simulink model "Symulacje"  (R2022a)
settings: Solver=VariableStepAuto  StartTime=0.0  StopTime=10000.0  RelTol=0.000001
undefined symbols (not defined in the file): aG1, aG2, aM1, aM2, aM3, aP1, aP2, aP3, bG1, bG2, bM1, bM2, bM3, bP1, bP2, bP3, cG1, cG2, cM1, cM2, cM3, cP1, cP2, cP3, DiscIntNeverNeededParam, KG1, KG2, KG3, KM1, KM2, KM3, KP1, KP2, KP3, kr1, kr2, kr3, T01, T02, T03, TG32, Ti1, Ti2, Ti3, Tzad1, Tzad2, Tzad3, waga1, waga2, waga3, waga4, waga5, waga6, waga7, waga8, waga9
libraries: simulink x15
settings Model: Creator=zawod  LastModifiedBy=zawod
settings SolverCC: ZeroCrossAlgorithm=Adaptive
settings DebuggingCC: AlgebraicLoopMsg=none  IgnoredZcDiagnostic=none

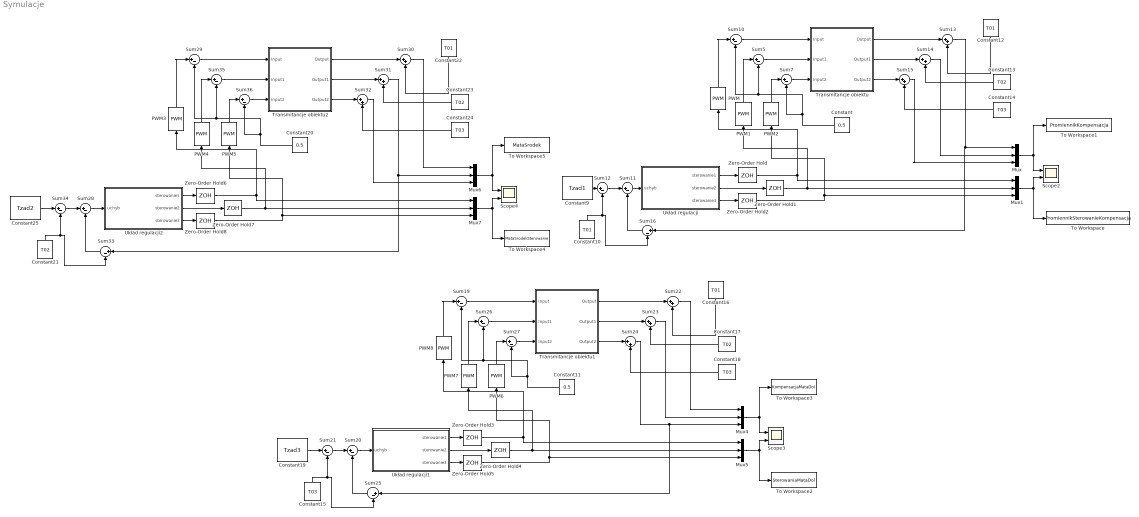
== system Symulacje ==
  Constant : Constant  Value=0.5
  Constant{10,12,16,22} (4 alike) : Constant  Value=T01
  Constant11 : Constant  Value=0.5
  Constant{13,17,21,23} (4 alike) : Constant  Value=T02
  Constant{14..15,18,24} (4 alike) : Constant  Value=T03
  Constant19 : Constant  Value=Tzad3
  Constant20 : Constant  Value=0.5
  Constant25 : Constant  Value=Tzad2
  Constant9 : Constant  Value=Tzad1
  Mux{,1,4..7} (6 alike) : Mux  Inputs=3
  PWM{,1..8} (9 alike) : simulink/Discontinuities/PWM  DisableCoverage=on  Period=10  DisallowZeroDutyCycle=off  RunAtFixedTimeIntervals=off  SampleTime=0.1
  Scope2 : Scope  NumInputPorts=2
  Scope3 : Scope  NumInputPorts=2
  Scope4 : Scope  NumInputPorts=2
  Sum{5,7,10..12,16,19..21,25..29,33..36} (18 alike) : Sum  Inputs=|+-
  Sum{13..15,22..24,30..32} (9 alike) : Sum  Inputs=|++
  To Workspace : ToWorkspace  VariableName=PromiennikSterowanieKompensacja  SaveFormat=Timeseries  SampleTime=-1
  To Workspace1 : ToWorkspace  VariableName=PromiennikKompensacja  SaveFormat=Timeseries  SampleTime=-1
  To Workspace2 : ToWorkspace  VariableName=SterowaniaMataDol  SaveFormat=Timeseries  SampleTime=-1
  To Workspace3 : ToWorkspace  VariableName=KompensacjaMataDol  SaveFormat=Timeseries  SampleTime=-1
  To Workspace4 : ToWorkspace  VariableName=MataSrodekSterowanie  SaveFormat=Timeseries  SampleTime=-1
  To Workspace5 : ToWorkspace  VariableName=MataSrodek  SaveFormat=Timeseries  SampleTime=-1
  Transmitancje obiektu : Subsystem
  Transmitancje obiektu1 : Subsystem
  Transmitancje obiektu2 : Subsystem
  Układ regulacji : Subsystem  mask{Kr=kr1, Ti=Ti1, Max=0.5, Min=-0.5}
      mask prompts: Kr "Kp"
  Układ regulacji1 : Subsystem  mask{Kr=kr3, Ti=Ti3, Max=0.5, Min=-0.5}
      mask prompts: Kr "Kp"
  Układ regulacji2 : Subsystem  mask{Kr=kr2, Ti=Ti2, Max=0.5, Min=-0.5}
      mask prompts: Kr "Kp"
  Zero-Order Hold{,1..8} (9 alike) : ZeroOrderHold  SampleTime=30
  wires:
  Transmitancje obiektu/3(Output2) -> Sum15/1
  Układ regulacji/3(sterowanie3) -> Zero-Order Hold2/1
  Constant/1 -> Sum10/2, Sum5/2, Sum7/2
  Constant9/1 -> Sum12/1
  Mux1/1 -> To Workspace/1, Scope2/2
  Constant13/1 -> Sum14/2
  Mux/1 -> Scope2/1, To Workspace1/1
  Układ regulacji/1(sterowanie1) -> Zero-Order Hold/1
  Układ regulacji/2(sterowanie2) -> Zero-Order Hold1/1
  Transmitancje obiektu/1(Output) -> Sum13/1
  Sum11/1 -> Układ regulacji/1(uchyb)
  Sum12/1 -> Sum11/1
  Constant12/1 -> Sum13/2
  Sum10/1 -> Transmitancje obiektu/1(Input)
  Constant10/1 -> Sum16/2, Sum12/2
  Sum16/1 -> Sum11/2
  Constant14/1 -> Sum15/2
  Transmitancje obiektu/2(Output1) -> Sum14/1
  Sum7/1 -> Transmitancje obiektu/3(Input2)
  Sum5/1 -> Transmitancje obiektu/2(Input1)
  Zero-Order Hold/1 -> PWM/1, Mux1/1
  Zero-Order Hold1/1 -> PWM1/1, Mux1/2
  Zero-Order Hold2/1 -> Mux1/3, PWM2/1
  Sum14/1 -> Mux/2
  Sum15/1 -> Mux/3
  Constant18/1 -> Sum24/2
  Sum20/1 -> Układ regulacji1/1(uchyb)
  Transmitancje obiektu1/2(Output1) -> Sum23/1
  Transmitancje obiektu1/3(Output2) -> Sum24/1
  Constant16/1 -> Sum22/2
  Sum27/1 -> Transmitancje obiektu1/3(Input2)
  Układ regulacji1/1(sterowanie1) -> Zero-Order Hold3/1
  Mux5/1 -> To Workspace2/1, Scope3/2
  Zero-Order Hold4/1 -> PWM7/1, Mux5/2
  Sum26/1 -> Transmitancje obiektu1/2(Input1)
  Zero-Order Hold3/1 -> PWM8/1, Mux5/1
  Sum22/1 -> Mux4/1
  Sum23/1 -> Mux4/2
  Constant15/1 -> Sum25/2, Sum21/2
  Sum19/1 -> Transmitancje obiektu1/1(Input)
  Constant11/1 -> Sum26/2, Sum19/2, Sum27/2
  Constant19/1 -> Sum21/1
  Constant17/1 -> Sum23/2
  Mux4/1 -> Scope3/1, To Workspace3/1
  Transmitancje obiektu1/1(Output) -> Sum22/1
  Układ regulacji1/3(sterowanie3) -> Zero-Order Hold5/1
  Zero-Order Hold5/1 -> Mux5/3, PWM6/1
  Sum25/1 -> Sum20/2
  Układ regulacji1/2(sterowanie2) -> Zero-Order Hold4/1
  Sum21/1 -> Sum20/1
  Sum30/1 -> Mux6/1
  Mux7/1 -> To Workspace4/1, Scope4/2
  Sum33/1 -> Sum28/2
  Mux6/1 -> Scope4/1, To Workspace5/1
  Constant22/1 -> Sum30/2
  Sum29/1 -> Transmitancje obiektu2/1(Input)
  Transmitancje obiektu2/3(Output2) -> Sum32/1
  Sum34/1 -> Sum28/1
  Constant24/1 -> Sum32/2
  Układ regulacji2/2(sterowanie2) -> Zero-Order Hold7/1
  Transmitancje obiektu2/2(Output1) -> Sum31/1
  Constant20/1 -> Sum35/2, Sum29/2, Sum36/2
  Transmitancje obiektu2/1(Output) -> Sum30/1
  Sum28/1 -> Układ regulacji2/1(uchyb)
  Zero-Order Hold6/1 -> PWM3/1, Mux7/1
  Sum35/1 -> Transmitancje obiektu2/2(Input1)
  Sum32/1 -> Mux6/3
  Układ regulacji2/3(sterowanie3) -> Zero-Order Hold8/1
  Sum36/1 -> Transmitancje obiektu2/3(Input2)
  Zero-Order Hold8/1 -> Mux7/3, PWM5/1
  Constant25/1 -> Sum34/1
  Constant23/1 -> Sum31/2
  Zero-Order Hold7/1 -> PWM4/1, Mux7/2
  Układ regulacji2/1(sterowanie1) -> Zero-Order Hold6/1
  Constant21/1 -> Sum33/2, Sum34/2
  PWM/1 -> Sum10/1
  PWM1/1 -> Sum5/1
  PWM2/1 -> Sum7/1
  Sum13/1 -> Sum16/1, Mux/1
  Sum24/1 -> Sum25/1, Mux4/3
  Sum31/1 -> Sum33/1, Mux6/2
  PWM3/1 -> Sum29/1
  PWM4/1 -> Sum35/1
  PWM5/1 -> Sum36/1
  PWM6/1 -> Sum27/1
  PWM7/1 -> Sum26/1
  PWM8/1 -> Sum19/1

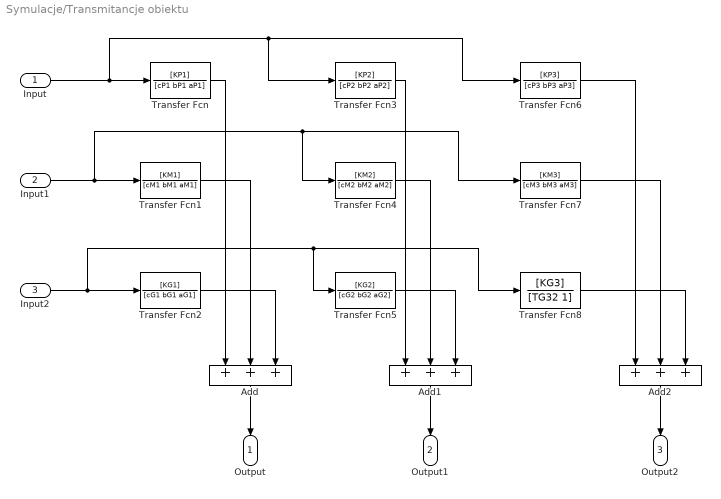
== system Symulacje/Transmitancje obiektu ==
  Input : Inport
  Input1 : Inport  Port=2
  Input2 : Inport  Port=3
  Add : Sum  Inputs=+++
  Add1 : Sum  Inputs=+++
  Add2 : Sum  Inputs=+++
  Transfer Fcn : TransferFcn  Numerator=[KP1]  Denominator=[cP1 bP1 aP1]
  Transfer Fcn1 : TransferFcn  Numerator=[KM1]  Denominator=[cM1 bM1 aM1]
  Transfer Fcn2 : TransferFcn  Numerator=[KG1]  Denominator=[cG1 bG1 aG1]
  Transfer Fcn3 : TransferFcn  Numerator=[KP2]  Denominator=[cP2 bP2 aP2]
  Transfer Fcn4 : TransferFcn  Numerator=[KM2]  Denominator=[cM2 bM2 aM2]
  Transfer Fcn5 : TransferFcn  Numerator=[KG2]  Denominator=[cG2 bG2 aG2]
  Transfer Fcn6 : TransferFcn  Numerator=[KP3]  Denominator=[cP3 bP3 aP3]
  Transfer Fcn7 : TransferFcn  Numerator=[KM3]  Denominator=[cM3 bM3 aM3]
  Transfer Fcn8 : TransferFcn  Numerator=[KG3]  Denominator=[TG32 1]
  Output : Outport
  Output1 : Outport  Port=2
  Output2 : Outport  Port=3
  wires:
  Input2/1 -> Transfer Fcn5/1, Transfer Fcn8/1, Transfer Fcn2/1
  Add1/1 -> Output1/1
  Transfer Fcn3/1 -> Add1/1
  Input1/1 -> Transfer Fcn7/1, Transfer Fcn4/1, Transfer Fcn1/1
  Transfer Fcn4/1 -> Add1/2
  Transfer Fcn8/1 -> Add2/3
  Transfer Fcn6/1 -> Add2/1
  Transfer Fcn5/1 -> Add1/3
  Add/1 -> Output/1
  Add2/1 -> Output2/1
  Transfer Fcn1/1 -> Add/2
  Transfer Fcn2/1 -> Add/3
  Input/1 -> Transfer Fcn6/1, Transfer Fcn3/1, Transfer Fcn/1
  Transfer Fcn/1 -> Add/1
  Transfer Fcn7/1 -> Add2/2

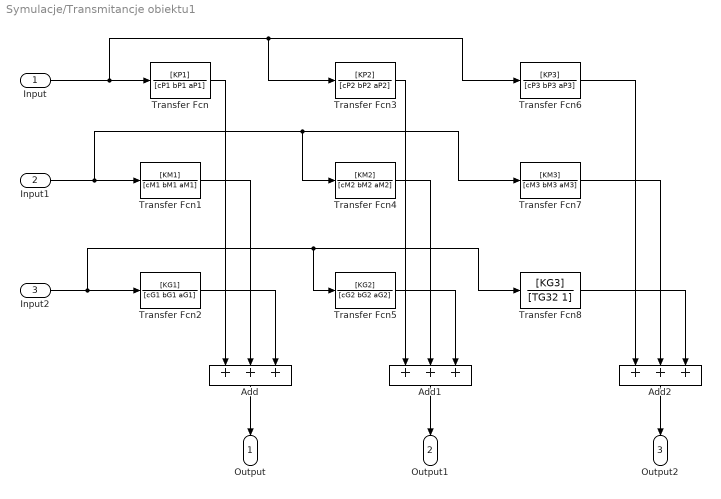
== system Symulacje/Transmitancje obiektu1 ==
  Input : Inport
  Input1 : Inport  Port=2
  Input2 : Inport  Port=3
  Add : Sum  Inputs=+++
  Add1 : Sum  Inputs=+++
  Add2 : Sum  Inputs=+++
  Transfer Fcn : TransferFcn  Numerator=[KP1]  Denominator=[cP1 bP1 aP1]
  Transfer Fcn1 : TransferFcn  Numerator=[KM1]  Denominator=[cM1 bM1 aM1]
  Transfer Fcn2 : TransferFcn  Numerator=[KG1]  Denominator=[cG1 bG1 aG1]
  Transfer Fcn3 : TransferFcn  Numerator=[KP2]  Denominator=[cP2 bP2 aP2]
  Transfer Fcn4 : TransferFcn  Numerator=[KM2]  Denominator=[cM2 bM2 aM2]
  Transfer Fcn5 : TransferFcn  Numerator=[KG2]  Denominator=[cG2 bG2 aG2]
  Transfer Fcn6 : TransferFcn  Numerator=[KP3]  Denominator=[cP3 bP3 aP3]
  Transfer Fcn7 : TransferFcn  Numerator=[KM3]  Denominator=[cM3 bM3 aM3]
  Transfer Fcn8 : TransferFcn  Numerator=[KG3]  Denominator=[TG32 1]
  Output : Outport
  Output1 : Outport  Port=2
  Output2 : Outport  Port=3
  wires:
  Input2/1 -> Transfer Fcn5/1, Transfer Fcn8/1, Transfer Fcn2/1
  Add1/1 -> Output1/1
  Transfer Fcn3/1 -> Add1/1
  Input1/1 -> Transfer Fcn7/1, Transfer Fcn4/1, Transfer Fcn1/1
  Transfer Fcn4/1 -> Add1/2
  Transfer Fcn8/1 -> Add2/3
  Transfer Fcn6/1 -> Add2/1
  Transfer Fcn5/1 -> Add1/3
  Add/1 -> Output/1
  Add2/1 -> Output2/1
  Transfer Fcn1/1 -> Add/2
  Transfer Fcn2/1 -> Add/3
  Input/1 -> Transfer Fcn6/1, Transfer Fcn3/1, Transfer Fcn/1
  Transfer Fcn/1 -> Add/1
  Transfer Fcn7/1 -> Add2/2

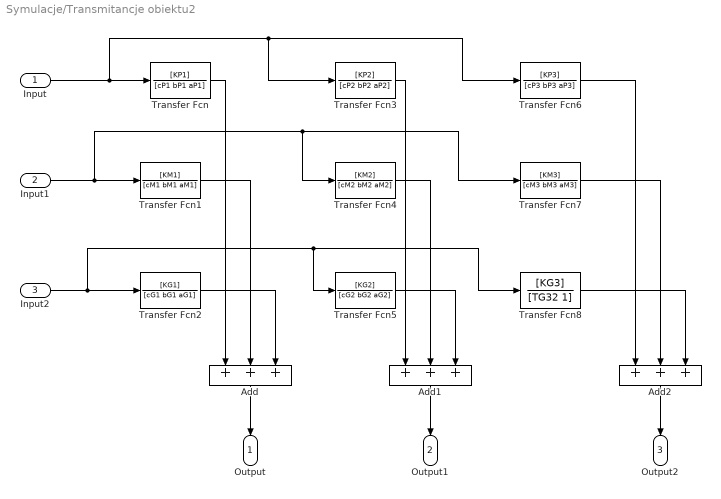
== system Symulacje/Transmitancje obiektu2 ==
  Input : Inport
  Input1 : Inport  Port=2
  Input2 : Inport  Port=3
  Add : Sum  Inputs=+++
  Add1 : Sum  Inputs=+++
  Add2 : Sum  Inputs=+++
  Transfer Fcn : TransferFcn  Numerator=[KP1]  Denominator=[cP1 bP1 aP1]
  Transfer Fcn1 : TransferFcn  Numerator=[KM1]  Denominator=[cM1 bM1 aM1]
  Transfer Fcn2 : TransferFcn  Numerator=[KG1]  Denominator=[cG1 bG1 aG1]
  Transfer Fcn3 : TransferFcn  Numerator=[KP2]  Denominator=[cP2 bP2 aP2]
  Transfer Fcn4 : TransferFcn  Numerator=[KM2]  Denominator=[cM2 bM2 aM2]
  Transfer Fcn5 : TransferFcn  Numerator=[KG2]  Denominator=[cG2 bG2 aG2]
  Transfer Fcn6 : TransferFcn  Numerator=[KP3]  Denominator=[cP3 bP3 aP3]
  Transfer Fcn7 : TransferFcn  Numerator=[KM3]  Denominator=[cM3 bM3 aM3]
  Transfer Fcn8 : TransferFcn  Numerator=[KG3]  Denominator=[TG32 1]
  Output : Outport
  Output1 : Outport  Port=2
  Output2 : Outport  Port=3
  wires:
  Input2/1 -> Transfer Fcn5/1, Transfer Fcn8/1, Transfer Fcn2/1
  Add1/1 -> Output1/1
  Transfer Fcn3/1 -> Add1/1
  Input1/1 -> Transfer Fcn7/1, Transfer Fcn4/1, Transfer Fcn1/1
  Transfer Fcn4/1 -> Add1/2
  Transfer Fcn8/1 -> Add2/3
  Transfer Fcn6/1 -> Add2/1
  Transfer Fcn5/1 -> Add1/3
  Add/1 -> Output/1
  Add2/1 -> Output2/1
  Transfer Fcn1/1 -> Add/2
  Transfer Fcn2/1 -> Add/3
  Input/1 -> Transfer Fcn6/1, Transfer Fcn3/1, Transfer Fcn/1
  Transfer Fcn/1 -> Add/1
  Transfer Fcn7/1 -> Add2/2

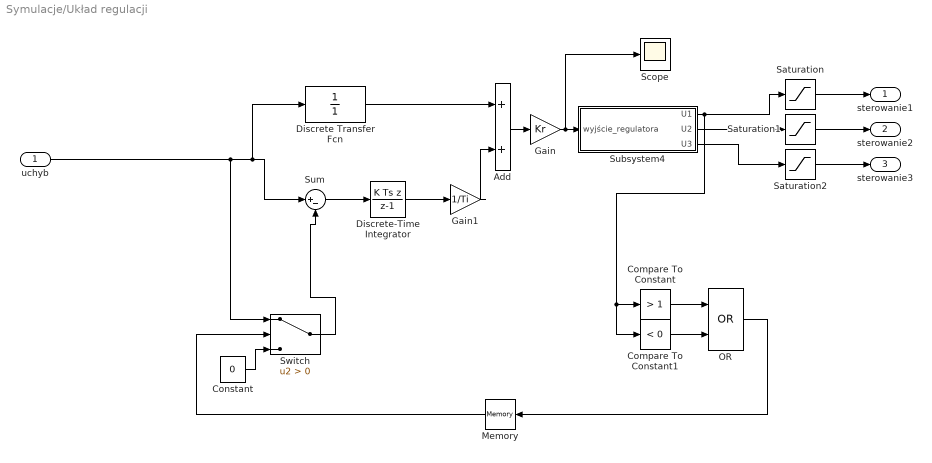
== system Symulacje/Układ regulacji ==
  uchyb : Inport
  Add : Sum
  Compare To Constant : simulink/Logic and Bit Operations/Compare To Constant  relop=>  const=1  OutDataTypeStr=uint8
  Compare To Constant1 : simulink/Logic and Bit Operations/Compare To Constant  relop=<  const=0  OutDataTypeStr=uint8
  Constant : Constant  Value=0
  Discrete Transfer Fcn : DiscreteTransferFcn  Denominator=[1]  SampleTime=30
  Discrete-Time Integrator : DiscreteIntegrator  IntegratorMethod=Integration: Backward Euler  SampleTime=30  ICPrevOutput=DiscIntNeverNeededParam  ICPrevScaledInput=DiscIntNeverNeededParam
  Gain : Gain  Gain=Kr
  Gain1 : Gain  Gain=1/Ti
  Memory : Memory
  OR : Logic  Operator=OR  IconShape=distinctive  AllPortsSameDT=off  OutDataTypeStr=boolean
  Saturation : Saturate  UpperLimit=1  LowerLimit=0
  Saturation1 : Saturate  UpperLimit=1  LowerLimit=0
  Saturation2 : Saturate  UpperLimit=1  LowerLimit=0
  Scope : Scope
  Subsystem4 : Subsystem
  Sum : Sum  Inputs=|+-
  Switch : Switch  Criteria=u2 > Threshold  SaturateOnIntegerOverflow=off  InputSameDT=off
  sterowanie1 : Outport
  sterowanie2 : Outport  Port=2
  sterowanie3 : Outport  Port=3
  wires:
  Gain1/1 -> Add/2
  Add/1 -> Gain/1
  Discrete-Time Integrator/1 -> Gain1/1
  Sum/1 -> Discrete-Time Integrator/1
  Switch/1 -> Sum/2
  Constant/1 -> Switch/3
  Subsystem4/2(U2) -> Saturation1/1
  Subsystem4/3(U3) -> Saturation2/1
  Subsystem4/1(U1) -> Saturation/1, Compare To Constant/1, Compare To Constant1/1
  Saturation/1 -> sterowanie1/1
  Saturation1/1 -> sterowanie2/1
  Saturation2/1 -> sterowanie3/1
  Compare To Constant/1 -> OR/1
  Compare To Constant1/1 -> OR/2
  Gain/1 -> Scope/1, Subsystem4/1(wyjście_regulatora)
  Memory/1 -> Switch/2
  uchyb/1 -> Sum/1, Discrete Transfer Fcn/1, Switch/1
  Discrete Transfer Fcn/1 -> Add/1
  OR/1 -> Memory/1

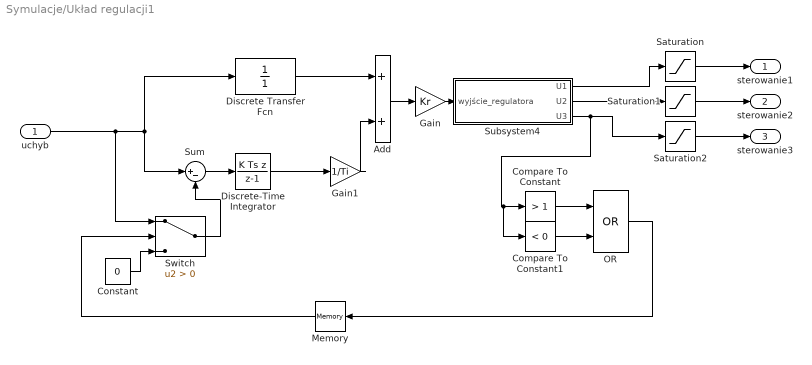
== system Symulacje/Układ regulacji1 ==
  uchyb : Inport
  Add : Sum
  Compare To Constant : simulink/Logic and Bit Operations/Compare To Constant  relop=>  const=1  OutDataTypeStr=boolean
  Compare To Constant1 : simulink/Logic and Bit Operations/Compare To Constant  relop=<  const=0  OutDataTypeStr=boolean
  Constant : Constant  Value=0
  Discrete Transfer Fcn : DiscreteTransferFcn  Denominator=[1]  SampleTime=30
  Discrete-Time Integrator : DiscreteIntegrator  IntegratorMethod=Integration: Backward Euler  SampleTime=30  ICPrevOutput=DiscIntNeverNeededParam  ICPrevScaledInput=DiscIntNeverNeededParam
  Gain : Gain  Gain=Kr
  Gain1 : Gain  Gain=1/Ti
  Memory : Memory
  OR : Logic  Operator=OR  IconShape=distinctive  AllPortsSameDT=off  OutDataTypeStr=boolean
  Saturation : Saturate  UpperLimit=1  LowerLimit=0
  Saturation1 : Saturate  UpperLimit=1  LowerLimit=0
  Saturation2 : Saturate  UpperLimit=1  LowerLimit=0
  Subsystem4 : Subsystem
  Sum : Sum  Inputs=|+-
  Switch : Switch  Criteria=u2 > Threshold  SaturateOnIntegerOverflow=off  InputSameDT=off
  sterowanie1 : Outport
  sterowanie2 : Outport  Port=2
  sterowanie3 : Outport  Port=3
  wires:
  Gain1/1 -> Add/2
  Add/1 -> Gain/1
  Discrete-Time Integrator/1 -> Gain1/1
  Sum/1 -> Discrete-Time Integrator/1
  Switch/1 -> Sum/2
  Constant/1 -> Switch/3
  Subsystem4/2(U2) -> Saturation1/1
  Subsystem4/3(U3) -> Compare To Constant1/1, Compare To Constant/1, Saturation2/1
  Gain/1 -> Subsystem4/1(wyjście_regulatora)
  Subsystem4/1(U1) -> Saturation/1
  Saturation/1 -> sterowanie1/1
  Saturation1/1 -> sterowanie2/1
  Saturation2/1 -> sterowanie3/1
  Compare To Constant/1 -> OR/1
  Compare To Constant1/1 -> OR/2
  OR/1 -> Memory/1
  uchyb/1 -> Switch/1, Sum/1, Discrete Transfer Fcn/1
  Memory/1 -> Switch/2
  Discrete Transfer Fcn/1 -> Add/1

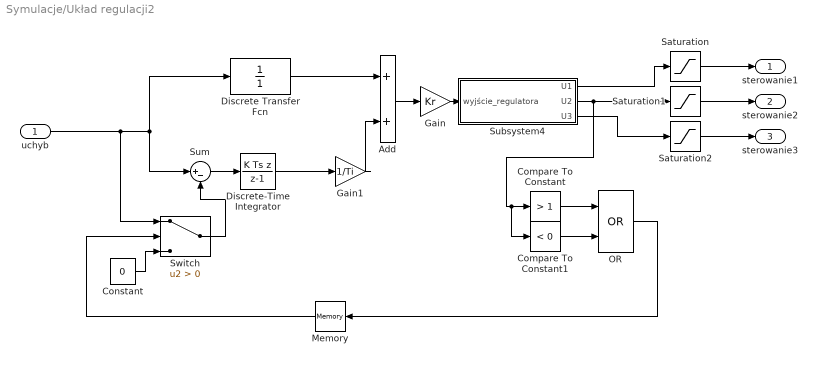
== system Symulacje/Układ regulacji2 ==
  uchyb : Inport
  Add : Sum
  Compare To Constant : simulink/Logic and Bit Operations/Compare To Constant  relop=>  const=1  OutDataTypeStr=boolean
  Compare To Constant1 : simulink/Logic and Bit Operations/Compare To Constant  relop=<  const=0  OutDataTypeStr=boolean
  Constant : Constant  Value=0
  Discrete Transfer Fcn : DiscreteTransferFcn  Denominator=[1]  SampleTime=30
  Discrete-Time Integrator : DiscreteIntegrator  IntegratorMethod=Integration: Backward Euler  SampleTime=30  ICPrevOutput=DiscIntNeverNeededParam  ICPrevScaledInput=DiscIntNeverNeededParam
  Gain : Gain  Gain=Kr
  Gain1 : Gain  Gain=1/Ti
  Memory : Memory
  OR : Logic  Operator=OR  IconShape=distinctive  AllPortsSameDT=off  OutDataTypeStr=boolean
  Saturation : Saturate  UpperLimit=1  LowerLimit=0
  Saturation1 : Saturate  UpperLimit=1  LowerLimit=0
  Saturation2 : Saturate  UpperLimit=1  LowerLimit=0
  Subsystem4 : Subsystem
  Sum : Sum  Inputs=|+-
  Switch : Switch  Criteria=u2 > Threshold  SaturateOnIntegerOverflow=off  InputSameDT=off
  sterowanie1 : Outport
  sterowanie2 : Outport  Port=2
  sterowanie3 : Outport  Port=3
  wires:
  Gain1/1 -> Add/2
  Add/1 -> Gain/1
  Discrete-Time Integrator/1 -> Gain1/1
  Sum/1 -> Discrete-Time Integrator/1
  Switch/1 -> Sum/2
  Constant/1 -> Switch/3
  Subsystem4/2(U2) -> Compare To Constant1/1, Compare To Constant/1, Saturation1/1
  Subsystem4/3(U3) -> Saturation2/1
  Gain/1 -> Subsystem4/1(wyjście_regulatora)
  Subsystem4/1(U1) -> Saturation/1
  Saturation/1 -> sterowanie1/1
  Saturation1/1 -> sterowanie2/1
  Saturation2/1 -> sterowanie3/1
  Compare To Constant/1 -> OR/1
  Compare To Constant1/1 -> OR/2
  OR/1 -> Memory/1
  uchyb/1 -> Switch/1, Sum/1, Discrete Transfer Fcn/1
  Memory/1 -> Switch/2
  Discrete Transfer Fcn/1 -> Add/1

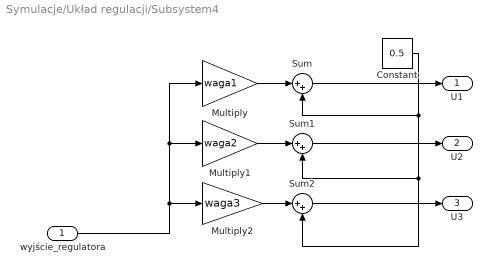
== system Symulacje/Układ regulacji/Subsystem4 ==
  wyjście_regulatora : Inport
  Constant : Constant  Value=0.5
  Multiply : Gain  Gain=waga1
  Multiply1 : Gain  Gain=waga2
  Multiply2 : Gain  Gain=waga3
  Sum : Sum  Inputs=|++
  Sum1 : Sum  Inputs=|++
  Sum2 : Sum  Inputs=|++
  U1 : Outport
  U2 : Outport  Port=2
  U3 : Outport  Port=3
  wires:
  wyjście_regulatora/1 -> Multiply/1, Multiply1/1, Multiply2/1
  Multiply/1 -> Sum/1
  Multiply1/1 -> Sum1/1
  Multiply2/1 -> Sum2/1
  Sum/1 -> U1/1
  Sum1/1 -> U2/1
  Sum2/1 -> U3/1
  Constant/1 -> Sum/2, Sum2/2, Sum1/2

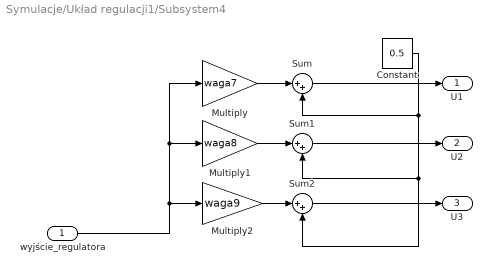
== system Symulacje/Układ regulacji1/Subsystem4 ==
  wyjście_regulatora : Inport
  Constant : Constant  Value=0.5
  Multiply : Gain  Gain=waga7
  Multiply1 : Gain  Gain=waga8
  Multiply2 : Gain  Gain=waga9
  Sum : Sum  Inputs=|++
  Sum1 : Sum  Inputs=|++
  Sum2 : Sum  Inputs=|++
  U1 : Outport
  U2 : Outport  Port=2
  U3 : Outport  Port=3
  wires:
  wyjście_regulatora/1 -> Multiply/1, Multiply1/1, Multiply2/1
  Multiply/1 -> Sum/1
  Multiply1/1 -> Sum1/1
  Multiply2/1 -> Sum2/1
  Sum/1 -> U1/1
  Sum1/1 -> U2/1
  Sum2/1 -> U3/1
  Constant/1 -> Sum/2, Sum2/2, Sum1/2

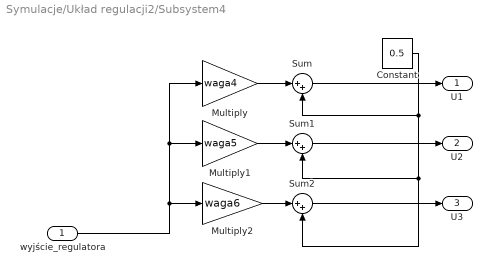
== system Symulacje/Układ regulacji2/Subsystem4 ==
  wyjście_regulatora : Inport
  Constant : Constant  Value=0.5
  Multiply : Gain  Gain=waga4
  Multiply1 : Gain  Gain=waga5
  Multiply2 : Gain  Gain=waga6
  Sum : Sum  Inputs=|++
  Sum1 : Sum  Inputs=|++
  Sum2 : Sum  Inputs=|++
  U1 : Outport
  U2 : Outport  Port=2
  U3 : Outport  Port=3
  wires:
  wyjście_regulatora/1 -> Multiply/1, Multiply1/1, Multiply2/1
  Multiply/1 -> Sum/1
  Multiply1/1 -> Sum1/1
  Multiply2/1 -> Sum2/1
  Sum/1 -> U1/1
  Sum1/1 -> U2/1
  Sum2/1 -> U3/1
  Constant/1 -> Sum/2, Sum2/2, Sum1/2
